simulink model "fxpdemo_sfun_user_dtprop"  (Simulink 5.0)
settings: Solver=FixedStepDiscrete  StartTime=0.0  StopTime=1  FixedStep=0.001  RelTol=1e-3
libraries: fixpt_lib_4 x4
settings Model: ExecutionOrder=on  Creator=andyb  LastModifiedBy=andyb  ExtModeAutoUpdateStatusClock=off  ParameterOverflowMsg=warning  ParameterPrecisionLossMsg=none  RTWInlineParameters=on  RTWOptions="-aEnforceIntegerDowncast=1 -aExtMode=0 -aExtModeTesting=0 -aFoldNonRolledExpr=1 -aForceParamTrailComments=0 -aGenerateComments=1 -aGenerateReport=1 -aIgnoreCustomStorageClasses=1 -aIncDataTypeInIds=0 -aIncHierarchyInIds=0 -aInlineInvariantSignals=0 -aInlineParameters=1 -aInlinedPrmAccess=\"Literals\" -aLocalBlockOutputs=1 -aLogVarNameModifier=\"rt_\" -aMaxRTWIdLen=31 -aPrefixModelToSubsysFcnNames=1 -aRTWVerbose=1 -aRollThreshold=5 -aShowEliminatedStatements=0"

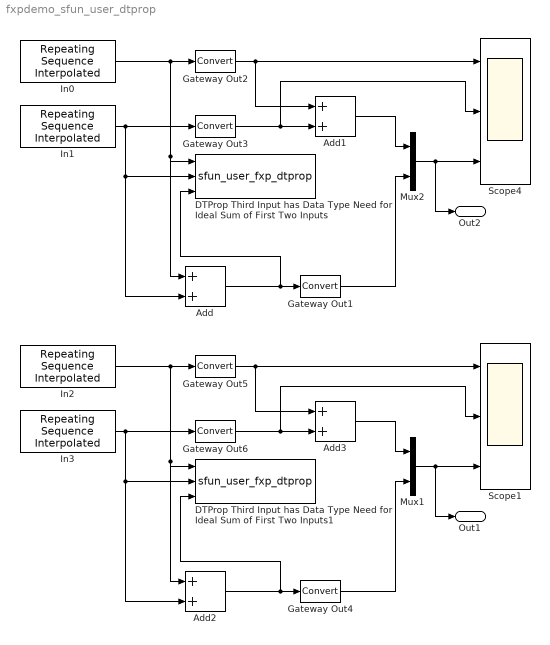
== system fxpdemo_sfun_user_dtprop ==
  Add : Sum  ShowAdditionalParam=on  OutScaling=2^-10
  Add1 : Sum  ShowAdditionalParam=on  OutDataTypeMode=double  OutScaling=2^-10
  Add2 : Sum  ShowAdditionalParam=on  OutScaling=2^-10
  Add3 : Sum  ShowAdditionalParam=on  OutDataTypeMode=double  OutScaling=2^-10
  DTProp Third Input has Data Type Need for Ideal Sum of First Two Inputs : S-Function  FunctionName=sfun_user_fxp_dtprop
  DTProp Third Input has Data Type Need for Ideal Sum of First Two Inputs1 : S-Function  FunctionName=sfun_user_fxp_dtprop
  Gateway Out{1..6} (6 alike) : DataTypeConversion  DataType=double
  In0 : fixpt_lib_4/Sources/Repeating Sequence Interpolated  OutValues=2^(16-1-8)*[-1 linspace(-1,0,5) 0 linspace(0,1,5) 1]  TimeValues=1/13*linspace(0,1,13)  LookUpMeth=Interpolation-Use End Values  tsamp=0.001  OutputDataTypeScalingMode=Specify via dialog  OutDataType=sfix(16)  OutScaling=2^-8
  In1 : fixpt_lib_4/Sources/Repeating Sequence Interpolated  OutValues=2^(16-1+(-5))*[-1 linspace(-1,0,5) 0 linspace(0,1,5) 1]  TimeValues=linspace(0,1,13)  LookUpMeth=Interpolation-Use End Values  tsamp=0.001  OutputDataTypeScalingMode=Specify via dialog  OutDataType=sfix(16)  OutScaling=2^-5
  In2 : fixpt_lib_4/Sources/Repeating Sequence Interpolated  OutValues=2^(5+(0))*[0 linspace(0,1,5) 1]  TimeValues=linspace(0,1,7)  LookUpMeth=Interpolation-Use End Values  tsamp=0.001  OutputDataTypeScalingMode=Specify via dialog  OutDataType=ufix(5)  OutScaling=2^0
  In3 : fixpt_lib_4/Sources/Repeating Sequence Interpolated  OutValues=2^(4+(-4))*[0 linspace(0,1,5) 1]  TimeValues=1/7*linspace(0,1,7)  LookUpMeth=Interpolation-Use End Values  tsamp=0.001  OutputDataTypeScalingMode=Specify via dialog  OutDataType=ufix(4)  OutScaling=2^-4
  Mux1 : Mux  Inputs=2
  Mux2 : Mux  Inputs=2
  Scope1 : Scope  NumInputPorts=3
      settings: TimeRange=1  YMin=0~0~0  YMax=35~1~35
  Scope4 : Scope  NumInputPorts=3
      settings: TimeRange=1  YMin=-150~-1500~-1500  YMax=150~1500~1500  SaveName=ScopeData3
  Out2 : Outport
  Out1 : Outport  Port=2
  wires:
  In1/1 -> Add/2, DTProp Third Input has Data Type Need for Ideal Sum of First Two Inputs/2, Gateway Out3/1
  Add/1 -> DTProp Third Input has Data Type Need for Ideal Sum of First Two Inputs/3, Gateway Out1/1
  Add1/1 -> Mux2/1
  Mux2/1 -> Scope4/3, Out2/1
  In0/1 -> Gateway Out2/1, DTProp Third Input has Data Type Need for Ideal Sum of First Two Inputs/1, Add/1
  Gateway Out3/1 -> Add1/2, Scope4/2
  Gateway Out2/1 -> Add1/1, Scope4/1
  Gateway Out1/1 -> Mux2/2
  In3/1 -> Gateway Out6/1, DTProp Third Input has Data Type Need for Ideal Sum of First Two Inputs1/2, Add2/2
  Add2/1 -> Gateway Out4/1, DTProp Third Input has Data Type Need for Ideal Sum of First Two Inputs1/3
  Add3/1 -> Mux1/1
  Mux1/1 -> Out1/1, Scope1/3
  In2/1 -> Add2/1, DTProp Third Input has Data Type Need for Ideal Sum of First Two Inputs1/1, Gateway Out5/1
  Gateway Out6/1 -> Scope1/2, Add3/2
  Gateway Out5/1 -> Scope1/1, Add3/1
  Gateway Out4/1 -> Mux1/2
